simulink model "RespiratorControl"  (R2018b)
settings: Solver=FixedStepDiscrete  StartTime=0.0  StopTime=30  FixedStep=MdlTS  RelTol=1e-3  EnableMultiTasking=on
libraries: LIB_Control x1
settings Model: DataDictionary=RespiratorControlData.sldd  Creator=BRAUL  LastModifiedBy=BRAUL
settings OptimizationCC: DefaultParameterBehavior=Inlined  UseFloatMulNetSlope=on  UseSpecifiedMinMax=on  InlineInvariantSignals=on  PassReuseOutputArgsAs=Individual arguments  ZeroExternalMemoryAtStartup=off  ZeroInternalMemoryAtStartup=off  NoFixptDivByZeroProtection=on  EfficientFloat2IntCast=on  LifeSpan=inf  MaxStackSize=64  OptimizeBlockOrder=speed  DifferentSizesBufferReuse=on
settings DebuggingCC: MergeDetectMultiDrivingBlocksExec=none  ParameterTunabilityLossMsg=error
settings HardwareCC: ProdBitPerPointer=32  ProdBitPerSizeT=32  ProdBitPerPtrDiffT=32  ProdLargestAtomicInteger=Long  ProdLargestAtomicFloat=Double  ProdWordSize=32  ProdLongLongMode=on  ProdHWDeviceType=ARM Compatible->ARM Cortex
settings ModelReferenceCC: ModelReferenceNumInstancesAllowed=Single  PropagateSignalLabelsOutOfModel=off
settings SFSimCC: MATLABDynamicMemAlloc=off
settings RTWCC: SystemTargetFile=ert.tlc  HardwareBoard=STM32 Nucleo F411RE  TemplateMakefile=ert_default_tmf  GenerateReport=on  Toolchain=GNU Tools for ARM Embedded Processors  BuildConfiguration=Faster Runs  IncludeHyperlinkInReport=on  LaunchReport=on  CodeExecutionProfiling=on  GenerateTraceInfo=on  GenerateTraceReport=on  GenerateTraceReportSl=on  GenerateTraceReportSf=on  GenerateTraceReportEml=on
settings CodeAppCC: ForceParamTrailComments=on  IgnoreCustomStorageClasses=off  OperatorAnnotations=on  SimulinkDataObjDesc=on  SFDataObjDesc=on  InsertBlockDesc=on
settings ERTTargetCC: TargetLangStandard=C99 (ISO)  CombineSignalStateStructs=on  SuppressErrorStatus=on  SupportNonFinite=off  SupportComplex=off

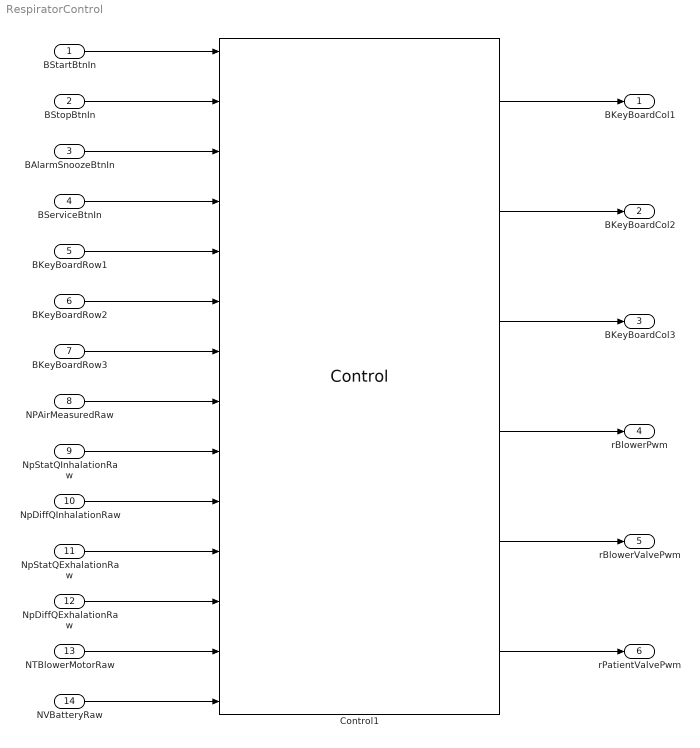
== system RespiratorControl ==
  BStartBtnIn : Inport  OutDataTypeStr=boolean
  BStopBtnIn : Inport  Port=2  OutDataTypeStr=boolean
  BAlarmSnoozeBtnIn : Inport  Port=3  OutDataTypeStr=boolean
  BServiceBtnIn : Inport  Port=4  OutDataTypeStr=boolean
  BKeyBoardRow1 : Inport  Port=5  OutDataTypeStr=boolean  PortDimensions=1
  BKeyBoardRow2 : Inport  Port=6  OutDataTypeStr=boolean  PortDimensions=1
  BKeyBoardRow3 : Inport  Port=7  OutDataTypeStr=boolean  PortDimensions=1
  NPAirMeasuredRaw : Inport  Port=8
  NpStatQInhalationRaw : Inport  Port=9  OutDataTypeStr=single
  NpDiffQInhalationRaw : Inport  Port=10  OutDataTypeStr=single
  NpStatQExhalationRaw : Inport  Port=11  OutDataTypeStr=single
  NpDiffQExhalationRaw : Inport  Port=12  OutDataTypeStr=single
  NTBlowerMotorRaw : Inport  Port=13
  NVBatteryRaw : Inport  Port=14
  Control1 : LIB_Control/Control  SystemSampleTime=-1
      settings: AttributesFormatString=%<ReferenceBlock>
  BKeyBoardCol1 : Outport  OutDataTypeStr=boolean  PortDimensions=1
  BKeyBoardCol2 : Outport  Port=2  OutDataTypeStr=boolean  PortDimensions=1
  BKeyBoardCol3 : Outport  Port=3  OutDataTypeStr=boolean  PortDimensions=1
  rBlowerPwm : Outport  Port=4  OutDataTypeStr=single
  rBlowerValvePwm : Outport  Port=5  OutDataTypeStr=single
  rPatientValvePwm : Outport  Port=6  OutDataTypeStr=single
  wires:
  NPAirMeasuredRaw/1 -> Control1/8
  Control1/4 -> rBlowerPwm/1
  Control1/5 -> rBlowerValvePwm/1
  Control1/6 -> rPatientValvePwm/1
  BServiceBtnIn/1 -> Control1/4
  BAlarmSnoozeBtnIn/1 -> Control1/3
  BStopBtnIn/1 -> Control1/2
  BStartBtnIn/1 -> Control1/1
  NTBlowerMotorRaw/1 -> Control1/13
  NVBatteryRaw/1 -> Control1/14
  BKeyBoardRow1/1 -> Control1/5
  BKeyBoardRow2/1 -> Control1/6
  BKeyBoardRow3/1 -> Control1/7
  Control1/1 -> BKeyBoardCol1/1
  Control1/2 -> BKeyBoardCol2/1
  Control1/3 -> BKeyBoardCol3/1
  NpStatQInhalationRaw/1 -> Control1/9
  NpDiffQInhalationRaw/1 -> Control1/10
  NpStatQExhalationRaw/1 -> Control1/11
  NpDiffQExhalationRaw/1 -> Control1/12
